simulink model "Verificacao_Controle_Pressao_2"  (R2018a)
settings: Solver=VariableStepAuto  StartTime=0.0  StopTime=60000  RelTol=1e-3
values from neighbouring files (symbols this model uses):
  alpha = Pacientes{i}('alpha')    [Analise_Exemplo.m]    (also in Analise_Geral_Robustez.m; Analise_Geral_Transitorio.m)
  Amplitude_perturbacao = 0    [Analise_Exemplo.m]    (also in Analise_Geral_Robustez.m = 25; Analise_Geral_Transitorio.m)
  ar = exp(-T/Constante_tempo_referencia)    [Analise_Exemplo.m]    (also in Analise_Geral_Robustez.m; Analise_Geral_Transitorio.m)
  ba_amplitude_seno = Pacientes{i}('ba_amplitude_seno')    [Analise_Exemplo.m]    (also in Analise_Geral_Robustez.m; Analise_Geral_Transitorio.m)
  ba_frequencia_seno = Pacientes{i}('ba_frequencia_seno')    [Analise_Exemplo.m]    (also in Analise_Geral_Robustez.m; Analise_Geral_Transitorio.m)
  ba_ganho_estocastico = Pacientes{i}('ba_ganho_estocastico')    [Analise_Exemplo.m]    (also in Analise_Geral_Robustez.m; Analise_Geral_Transitorio.m)
  ba_limiar_reflexo = Pacientes{i}('ba_limiar_reflexo')    [Analise_Exemplo.m]    (also in Analise_Geral_Robustez.m; Analise_Geral_Transitorio.m)
  ba_offset = Pacientes{i}('ba_offset')    [Analise_Exemplo.m]    (also in Analise_Geral_Robustez.m; Analise_Geral_Transitorio.m)
  comando_inicial = 0    [Analise_Exemplo.m]    (also in Analise_Geral_Robustez.m; Analise_Geral_Transitorio.m)
  d = 5    [Analise_Exemplo.m]    (also in Analise_Geral_Robustez.m; Analise_Geral_Transitorio.m)
  forgetting_factor = exp(-T/T_forgetting)    [Analise_Exemplo.m]    (also in Analise_Geral_Robustez.m; Analise_Geral_Transitorio.m)
  Instante_habilita_controlador = 30    [Analise_Exemplo.m]    (also in Analise_Geral_Robustez.m; Analise_Geral_Transitorio.m)
  Instante_habilita_perturbacao = 3*60*60    (= 10800)    [Analise_Exemplo.m]    (also in Analise_Geral_Robustez.m; Analise_Geral_Transitorio.m)
  K = Pacientes{i}('K')    [Analise_Exemplo.m]    (also in Analise_Geral_Robustez.m; Analise_Geral_Transitorio.m)
  P_inicial = [0.01 0 0; 0 0.001 0 ; 0 0 1]    [Analise_Exemplo.m]    (also in Analise_Geral_Robustez.m; Analise_Geral_Transitorio.m)
  saida_inicial_maxima = 0    [Analise_Exemplo.m]    (also in Analise_Geral_Robustez.m; Analise_Geral_Transitorio.m)
  semente_ruido = 2    [Analise_Exemplo.m]    (also in Analise_Geral_Robustez.m = j; Analise_Geral_Transitorio.m = j)
  setpoint_final = 116    [Analise_Exemplo.m]    (also in Analise_Geral_Robustez.m = 120; Analise_Geral_Transitorio.m)
  setpoint_inicial = 131    [Analise_Exemplo.m]    (also in Analise_Geral_Robustez.m = 150; Analise_Geral_Transitorio.m)
  T = 15    [Analise_Exemplo.m]    (also in Analise_Geral_Robustez.m; Analise_Geral_Transitorio.m)
  Tau = Pacientes{i}('Tau')    [Analise_Exemplo.m]    (also in Analise_Geral_Robustez.m; Analise_Geral_Transitorio.m)
  Tau_c = Pacientes{i}('Tau_c')    [Analise_Exemplo.m]    (also in Analise_Geral_Robustez.m; Analise_Geral_Transitorio.m)
  Tau_i = Pacientes{i}('Tau_i');5    [Analise_Exemplo.m]    (also in Analise_Geral_Robustez.m; Analise_Geral_Transitorio.m)
  Tempo_Segundo_Step = 30*60    (= 1800)    [Analise_Exemplo.m]    (also in Analise_Geral_Robustez.m; Analise_Geral_Transitorio.m)
  theta_inicial = [c0_inicial; c1_inicial; c2_inicial]    [Analise_Exemplo.m]    (also in Analise_Geral_Robustez.m; Analise_Geral_Transitorio.m)
libraries: simulink x1, powerlib_meascontrol x1
settings Model: Creator=gabri  LastModifiedBy=gabri

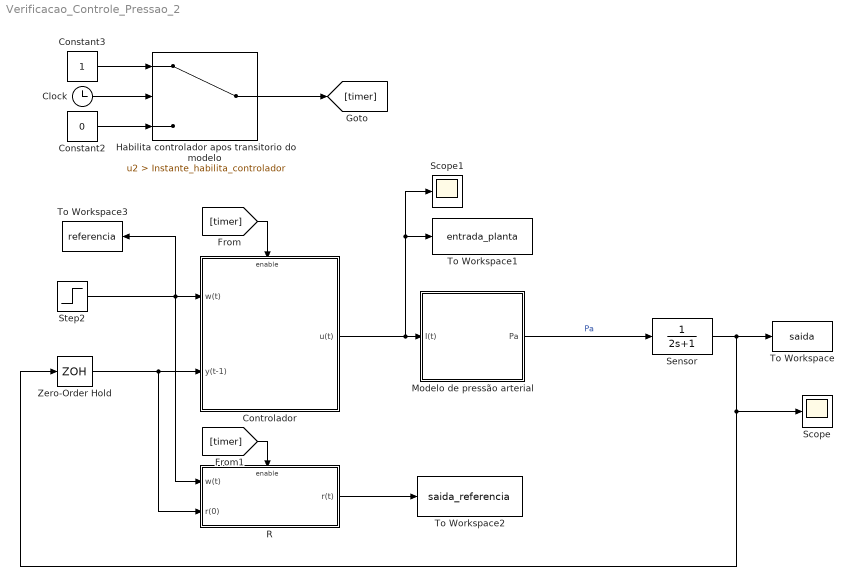
== system Verificacao_Controle_Pressao_2 ==
  Clock : Clock
  Constant2 : Constant  Value=0
  Constant3 : Constant
  "Controlador " : Subsystem
  Habilita controlador apos transitorio do modelo : Switch  Criteria=u2 > Threshold  Threshold=Instante_habilita_controlador  ZeroCross=off
  Modelo de pressão arterial : Subsystem
  R : Subsystem  TreatAsAtomicUnit=on
  Scope : Scope
  Scope1 : Scope
  Sensor : TransferFcn  Denominator=[2 1]
  Step2 : Step  Time=Instante_habilita_controlador+Tempo_Segundo_Step  Before=setpoint_inicial  After=setpoint_final  SampleTime=0
  To Workspace : ToWorkspace  VariableName=saida  SaveFormat=Timeseries  SampleTime=-1
  To Workspace1 : ToWorkspace  VariableName=entrada_planta  SaveFormat=Timeseries  SampleTime=-1
  To Workspace2 : ToWorkspace  VariableName=saida_referencia  SaveFormat=Timeseries  SampleTime=-1
  To Workspace3 : ToWorkspace  VariableName=referencia  SaveFormat=Timeseries  SampleTime=-1
  Zero-Order Hold : ZeroOrderHold  SampleTime=T
  wires:
  Constant2/1 -> Habilita controlador apos transitorio do modelo/3
  Habilita controlador apos transitorio do modelo/1 -> [timer]
  Clock/1 -> Habilita controlador apos transitorio do modelo/2
  Constant3/1 -> Habilita controlador apos transitorio do modelo/1
  Modelo de pressão arterial/1(Pa) -> Sensor/1  "Pa"
  [timer] -> "Controlador "/Enable
  R/1(r(t)) -> To Workspace2/1
  [timer] -> R/Enable
  Zero-Order Hold/1 -> R/2(r(0)), "Controlador "/2(y(t-1))
  "Controlador "/1(u(t)) -> Modelo de pressão arterial/1(I(t)), Scope1/1, To Workspace1/1
  Sensor/1 -> To Workspace/1, Scope/1, Zero-Order Hold/1
  Step2/1 -> R/1(w(t)), To Workspace3/1, "Controlador "/1(w(t))

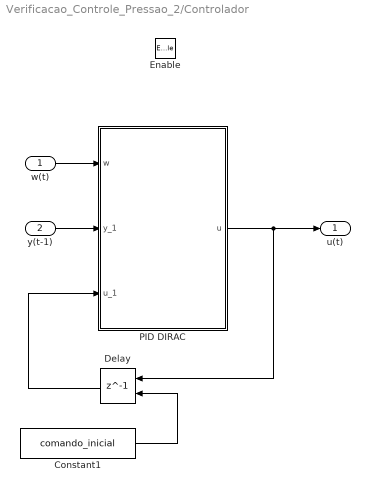
== system Verificacao_Controle_Pressao_2/Controlador  ==
  w(t) : Inport
  y(t-1) : Inport  Port=2
  Enable : EnablePort
  Constant1 : Constant  Value=comando_inicial
  Delay : Delay  DelayLength=1  InitialConditionSource=Input port  InitialCondition=0  SampleTime=T
      settings: InputPortMap=u0,p4
  PID DIRAC : Subsystem
  u(t) : Outport
  wires:
  w(t)/1 -> PID DIRAC/1("w ")
  Delay/1 -> PID DIRAC/3(u_1)
  y(t-1)/1 -> PID DIRAC/2(y_1)
  Constant1/1 -> Delay/2
  PID DIRAC/1(u) -> u(t)/1, Delay/1

== system Verificacao_Controle_Pressao_2/Modelo de pressão arterial ==
  I(t) : Inport
  Add : Sum
  Atividade de Background : Subsystem
  Resposta ao medicamento : Subsystem
  Pa : Outport
  wires:
  Resposta ao medicamento/1(Delta_Pd) -> Add/1
  I(t)/1 -> Resposta ao medicamento/1(I)
  Add/1 -> Pa/1, Atividade de Background/1(pa)  "Pa"
  Atividade de Background/1("Background Offset ") -> Add/2

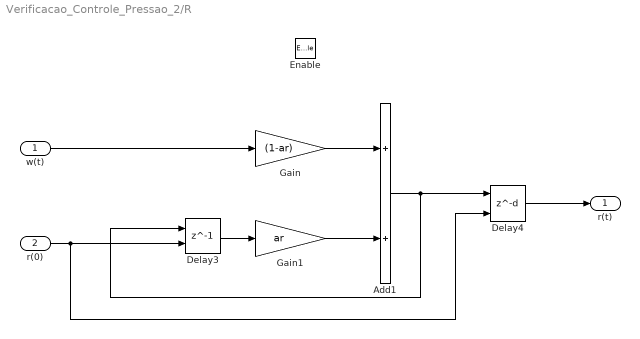
== system Verificacao_Controle_Pressao_2/R ==
  w(t) : Inport
  r(0) : Inport  Port=2
  Enable : EnablePort
  Add1 : Sum
  Delay3 : Delay  DelayLength=1  InitialConditionSource=Input port  InitialCondition=100  SampleTime=T
      settings: InputPortMap=u0,p4
  Delay4 : Delay  DelayLength=d  InitialConditionSource=Input port  InitialCondition=0  SampleTime=T
      settings: InputPortMap=u0,p4
  Gain : Gain  Gain=(1-ar)
  Gain1 : Gain  Gain=ar
  r(t) : Outport
  wires:
  Delay3/1 -> Gain1/1
  w(t)/1 -> Gain/1
  Gain1/1 -> Add1/2
  Gain/1 -> Add1/1
  r(0)/1 -> Delay4/2, Delay3/2
  Add1/1 -> Delay4/1, Delay3/1
  Delay4/1 -> r(t)/1

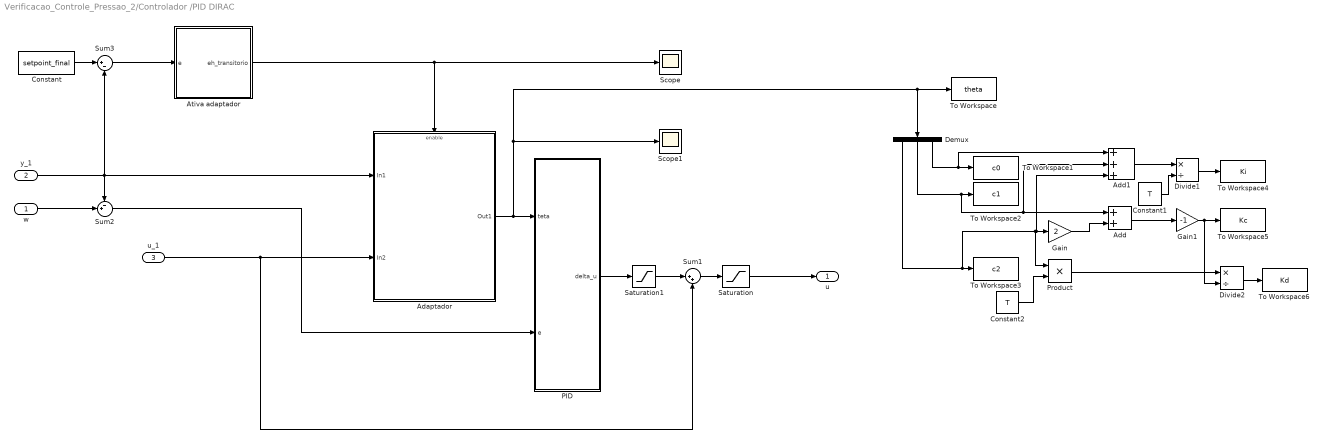
== system Verificacao_Controle_Pressao_2/Controlador /PID DIRAC ==
  "w " : Inport
  y_1 : Inport  Port=2
  u_1 : Inport  Port=3
  Adaptador : Subsystem
  Add : Sum
  Add1 : Sum  Inputs=+++
  Ativa adaptador : Subsystem
  Constant : Constant  Value=setpoint_final
  Constant1 : Constant  Value=T
  Constant2 : Constant  Value=T
  Demux : Demux  Outputs=3
  Divide1 : Product  Inputs=*/
  Divide2 : Product  Inputs=*/
  Gain : Gain  Gain=2
  Gain1 : Gain  Gain=-1
  PID : Subsystem
  Product : Product
  Saturation : Saturate  UpperLimit=180  LowerLimit=0
  Saturation1 : Saturate  UpperLimit=3  LowerLimit=-40
  Scope : Scope
  Scope1 : Scope
  Sum1 : Sum  Inputs=|++
  Sum2 : Sum  Inputs=-+|
  Sum3 : Sum  Inputs=|+-
  To Workspace : ToWorkspace  VariableName=theta  SaveFormat=Timeseries  SampleTime=-1
  To Workspace1 : ToWorkspace  VariableName=c0  SaveFormat=Timeseries  SampleTime=-1
  To Workspace2 : ToWorkspace  VariableName=c1  SaveFormat=Timeseries  SampleTime=-1
  To Workspace3 : ToWorkspace  VariableName=c2  SaveFormat=Timeseries  SampleTime=-1
  To Workspace4 : ToWorkspace  VariableName=Ki  SaveFormat=Timeseries  SampleTime=-1
  To Workspace5 : ToWorkspace  VariableName=Kc  SaveFormat=Timeseries  SampleTime=-1
  To Workspace6 : ToWorkspace  VariableName=Kd  SaveFormat=Timeseries  SampleTime=-1
  u : Outport
  wires:
  PID/1(delta_u) -> Saturation1/1
  Sum1/1 -> Saturation/1
  Saturation1/1 -> Sum1/1
  Saturation/1 -> u/1
  Sum2/1 -> PID/2(e)
  "w "/1 -> Sum2/2
  u_1/1 -> Sum1/2, Adaptador/2(In2)
  Constant/1 -> Sum3/1
  y_1/1 -> Adaptador/1(In1), Sum3/2, Sum2/1
  Ativa adaptador/1(eh_transitorio) -> Adaptador/Enable, Scope/1
  Sum3/1 -> Ativa adaptador/1(e)
  Demux/3 -> Add1/1, To Workspace1/1
  Demux/1 -> Product/1, Add1/3, Gain/1, To Workspace3/1
  Demux/2 -> Add1/2, Add/1, To Workspace2/1
  Adaptador/1(Out1) -> Scope1/1, To Workspace/1, Demux/1, PID/1(teta)
  Gain/1 -> Add/2
  Add/1 -> Gain1/1
  Add1/1 -> Divide1/1
  Constant1/1 -> Divide1/2
  Constant2/1 -> Product/2
  Product/1 -> Divide2/1
  Divide1/1 -> To Workspace4/1
  Gain1/1 -> Divide2/2, To Workspace5/1
  Divide2/1 -> To Workspace6/1

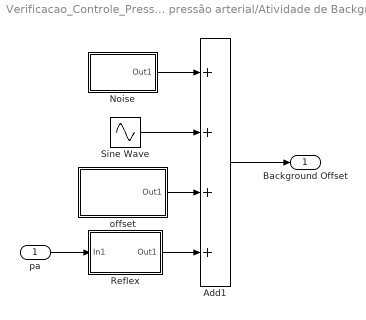
== system Verificacao_Controle_Pressao_2/Modelo de pressão arterial/Atividade de Background ==
  pa : Inport
  Add1 : Sum  Inputs=++++
  "Noise " : Subsystem
  Reflex : Subsystem
  Sine Wave : Sin  Amplitude=ba_amplitude_seno  Frequency=ba_frequencia_seno  SampleTime=0
  offset : Subsystem
  "Background Offset " : Outport
  wires:
  Reflex/1(Out1) -> Add1/4
  Add1/1 -> "Background Offset "/1
  "Noise "/1(Out1) -> Add1/1
  Sine Wave/1 -> Add1/2
  pa/1 -> Reflex/1(In1)
  offset/1(Out1) -> Add1/3

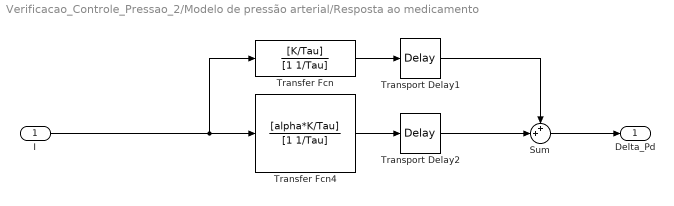
== system Verificacao_Controle_Pressao_2/Modelo de pressão arterial/Resposta ao medicamento ==
  I : Inport
  Sum : Sum  Inputs=++|
  Transfer Fcn : TransferFcn  Numerator=[K/Tau]  Denominator=[1 1/Tau]
  Transfer Fcn4 : TransferFcn  Numerator=[alpha*K/Tau]  Denominator=[1 1/Tau]
  Transport Delay1 : TransportDelay  DelayTime=Tau_i
  Transport Delay2 : TransportDelay  DelayTime=Tau_i+Tau_c
  Delta_Pd : Outport
  wires:
  Transport Delay1/1 -> Sum/1
  I/1 -> Transfer Fcn/1, Transfer Fcn4/1
  Transfer Fcn/1 -> Transport Delay1/1
  Transfer Fcn4/1 -> Transport Delay2/1
  Transport Delay2/1 -> Sum/2
  Sum/1 -> Delta_Pd/1

== system Verificacao_Controle_Pressao_2/Controlador /PID DIRAC/Adaptador ==
  In1 : Inport
  In2 : Inport  Port=2
  Enable : EnablePort
  Estimador2 : Subsystem
  Interface do Estimador : Subsystem
  Out1 : Outport
  wires:
  In1/1 -> Interface do Estimador/1("yf(t) ")
  Estimador2/1(theta) -> Out1/1
  Interface do Estimador/1("psi ") -> Estimador2/1(psi)
  Interface do Estimador/2(phi) -> Estimador2/2(phi)
  In2/1 -> Interface do Estimador/2(uf(t))

== system Verificacao_Controle_Pressao_2/Controlador /PID DIRAC/Ativa adaptador ==
  e : Inport
  Constant1 : Constant  Value=0
  Constant3 : Constant
  Is accomodated after rising : Subsystem
  Switch1 : Switch  Threshold=1
  eh_transitorio : Outport
  wires:
  Switch1/1 -> eh_transitorio/1
  e/1 -> Is accomodated after rising/1(In1)
  Is accomodated after rising/1(Out1) -> Switch1/2
  Constant3/1 -> Switch1/3
  Constant1/1 -> Switch1/1

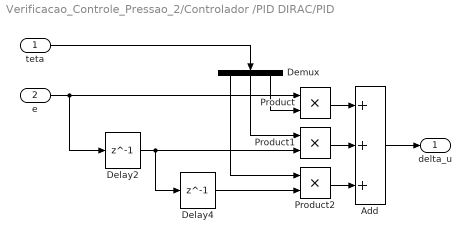
== system Verificacao_Controle_Pressao_2/Controlador /PID DIRAC/PID ==
  teta : Inport
  e : Inport  Port=2
  Add : Sum  Inputs=+++
  Delay2 : Delay  DelayLength=1  InitialCondition=0  SampleTime=T
  Delay4 : Delay  DelayLength=1  InitialCondition=0  SampleTime=T
  Demux : Demux  Outputs=3
  Product : Product
  Product1 : Product
  Product2 : Product
  delta_u : Outport
  wires:
  teta/1 -> Demux/1
  Delay2/1 -> Product1/2, Delay4/1
  Delay4/1 -> Product2/2
  Add/1 -> delta_u/1
  Demux/3 -> Product/2
  Demux/2 -> Product1/1
  Demux/1 -> Product2/1
  Product/1 -> Add/1
  Product1/1 -> Add/2
  Product2/1 -> Add/3
  e/1 -> Delay2/1, Product/1

== system Verificacao_Controle_Pressao_2/Modelo de pressão arterial/Atividade de Background/Noise  ==
  Random Number : RandomNumber  Seed=semente_ruido  SampleTime=T
  Saturation : Saturate  UpperLimit=ba_ganho_estocastico  LowerLimit=-ba_ganho_estocastico
  Transfer Fcn : TransferFcn  Numerator=[ba_ganho_estocastico]  Denominator=[30^2 2*30 1]
  Out1 : Outport
  wires:
  Transfer Fcn/1 -> Saturation/1
  Random Number/1 -> Transfer Fcn/1
  Saturation/1 -> Out1/1

== system Verificacao_Controle_Pressao_2/Modelo de pressão arterial/Atividade de Background/Reflex ==
  In1 : Inport
  Add2 : Sum  Inputs=-+
  Constant2 : Constant  Value=ba_limiar_reflexo
  Saturation : Saturate  UpperLimit=0  LowerLimit=-35
  Transfer Fcn2 : TransferFcn  Denominator=[240 1]
  Transport Delay : TransportDelay  DelayTime=40
  Out1 : Outport
  wires:
  Saturation/1 -> Transport Delay/1
  In1/1 -> Add2/2
  Transport Delay/1 -> Transfer Fcn2/1
  Constant2/1 -> Add2/1
  Add2/1 -> Saturation/1
  Transfer Fcn2/1 -> Out1/1

== system Verificacao_Controle_Pressao_2/Modelo de pressão arterial/Atividade de Background/offset ==
  Constant2 : Constant  Value=ba_offset
  Step : Step  Time=Instante_habilita_perturbacao  After=Amplitude_perturbacao  SampleTime=0
  Sum1 : Sum  Inputs=++|
  To Workspace : ToWorkspace  VariableName=atividade_background  SaveFormat=Timeseries  SampleTime=-1
  Out1 : Outport
  wires:
  Constant2/1 -> Sum1/1
  Step/1 -> Sum1/2
  Sum1/1 -> To Workspace/1, Out1/1

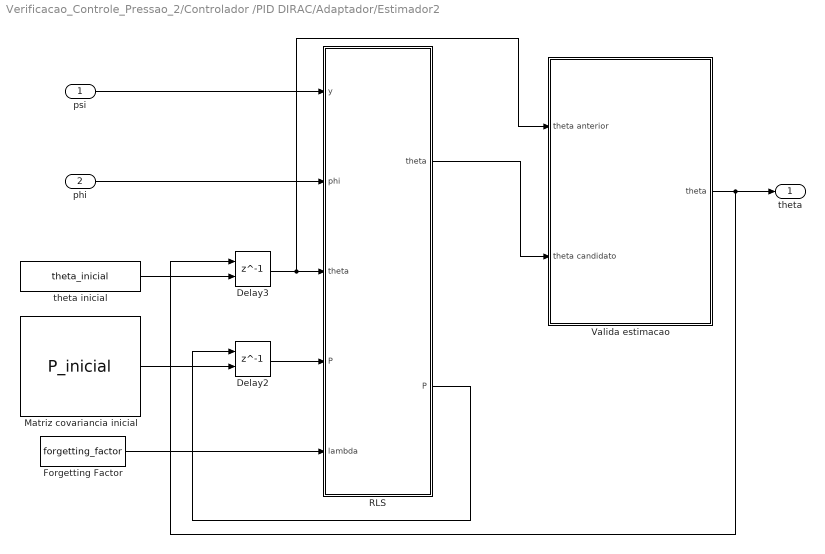
== system Verificacao_Controle_Pressao_2/Controlador /PID DIRAC/Adaptador/Estimador2 ==
  psi : Inport
  phi : Inport  Port=2
  Delay2 : Delay  DelayLength=1  InitialConditionSource=Input port  InitialCondition=0  SampleTime=T
      settings: InputPortMap=u0,p4
  Delay3 : Delay  DelayLength=1  InitialConditionSource=Input port  InitialCondition=0  SampleTime=T
      settings: InputPortMap=u0,p4
  Forgetting Factor : Constant  Value=forgetting_factor
  Matriz covariancia inicial : Constant  Value=P_inicial
  RLS : MATLAB Function  TreatAsAtomicUnit=on
  Valida estimacao : Subsystem
  theta inicial : Constant  Value=theta_inicial
  theta : Outport
  wires:
  Delay3/1 -> Valida estimacao/1(theta anterior), RLS/3("theta ")
  RLS/1(theta) -> Valida estimacao/2(theta candidato)
  Valida estimacao/1(theta) -> Delay3/1, theta/1
  Forgetting Factor/1 -> RLS/5(lambda)
  psi/1 -> RLS/1(y)
  RLS/2(P) -> Delay2/1
  theta inicial/1 -> Delay3/2
  phi/1 -> RLS/2(phi)
  Delay2/1 -> RLS/4("P ")
  Matriz covariancia inicial/1 -> Delay2/2

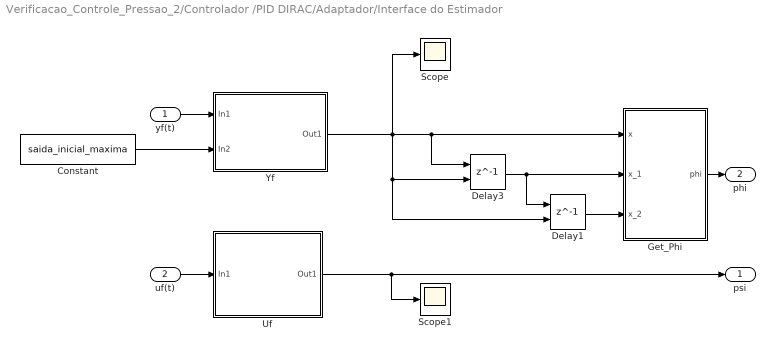
== system Verificacao_Controle_Pressao_2/Controlador /PID DIRAC/Adaptador/Interface do Estimador ==
  "yf(t) " : Inport
  uf(t) : Inport  Port=2
  Constant : Constant  Value=saida_inicial_maxima
  Delay1 : Delay  DelayLength=1  InitialConditionSource=Input port  InitialCondition=0  SampleTime=T
      settings: InputPortMap=u0,p4
  Delay3 : Delay  DelayLength=1  InitialConditionSource=Input port  InitialCondition=0  SampleTime=T
      settings: InputPortMap=u0,p4
  "Get_Phi " : MATLAB Function  TreatAsAtomicUnit=on
  Scope : Scope
  Scope1 : Scope
  Uf : Subsystem
  Yf : Subsystem
  "psi " : Outport
  phi : Outport  Port=2
  wires:
  Delay1/1 -> "Get_Phi "/3(x_2)
  Delay3/1 -> "Get_Phi "/2(x_1), Delay1/1
  "Get_Phi "/1(phi) -> phi/1
  Yf/1(Out1) -> Delay1/2, Delay3/2, Scope/1, Delay3/1, "Get_Phi "/1(x)
  Uf/1(Out1) -> Scope1/1, "psi "/1
  Constant/1 -> Yf/2(In2)
  "yf(t) "/1 -> Yf/1(In1)
  uf(t)/1 -> Uf/1(In1)

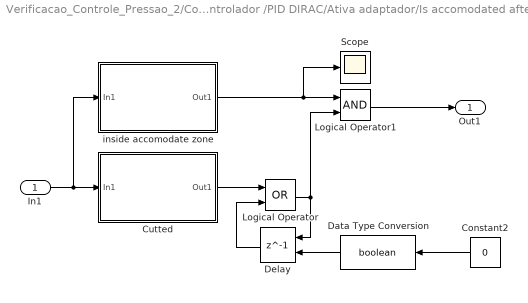
== system Verificacao_Controle_Pressao_2/Controlador /PID DIRAC/Ativa adaptador/Is accomodated after rising ==
  In1 : Inport
  Constant2 : Constant  Value=0
  Cutted : Subsystem
  Data Type Conversion : DataTypeConversion  OutDataTypeStr=boolean
  Delay : Delay  DelayLength=1  InitialConditionSource=Input port  InitialCondition=0
      settings: InputPortMap=u0,p4
  Logical Operator : Logic  Operator=OR  AllPortsSameDT=off  OutDataTypeStr=boolean
  Logical Operator1 : Logic  AllPortsSameDT=off  OutDataTypeStr=boolean
  Scope : Scope
  inside accomodate zone : Subsystem
  Out1 : Outport
  wires:
  inside accomodate zone/1(Out1) -> Scope/1, Logical Operator1/1
  Logical Operator/1 -> Logical Operator1/2, Delay/1
  Constant2/1 -> Data Type Conversion/1
  Logical Operator1/1 -> Out1/1
  In1/1 -> inside accomodate zone/1(In1), Cutted/1(In1)
  Cutted/1(Out1) -> Logical Operator/1
  Delay/1 -> Logical Operator/2
  Data Type Conversion/1 -> Delay/2

== system Verificacao_Controle_Pressao_2/Controlador /PID DIRAC/Adaptador/Estimador2/Valida estimacao ==
  theta anterior : Inport
  theta candidato : Inport  Port=2
  Compare To Zero : simulink/Logic and Bit Operations/Compare To Zero  relop=<=  OutDataTypeStr=boolean
  Switch2 : Switch  Criteria=u2 > Threshold
  Valida Estimacao : MATLAB Function  TreatAsAtomicUnit=on
  theta : Outport
  wires:
  Switch2/1 -> theta/1
  Compare To Zero/1 -> Switch2/2
  theta anterior/1 -> Switch2/3
  Valida Estimacao/1(eh_invalido) -> Compare To Zero/1
  theta candidato/1 -> Switch2/1, Valida Estimacao/1(theta_candidato)

== system Verificacao_Controle_Pressao_2/Controlador /PID DIRAC/Adaptador/Interface do Estimador/Uf ==
  In1 : Inport
  Delay2 : Delay  DelayLength=1
  R : Subsystem  TreatAsAtomicUnit=on
  Sum3 : Sum  Inputs=|+-
  Out1 : Outport
  wires:
  R/1(r(t)) -> Sum3/1, Delay2/1
  Delay2/1 -> Sum3/2
  Sum3/1 -> Out1/1
  In1/1 -> R/2(r(0)), R/1(w(t))

== system Verificacao_Controle_Pressao_2/Controlador /PID DIRAC/Adaptador/Interface do Estimador/Yf ==
  In1 : Inport
  In2 : Inport  Port=2
  R : Subsystem  TreatAsAtomicUnit=on
  Sum2 : Sum  Inputs=|+-
  Sum4 : Sum  Inputs=|-+
  Out1 : Outport
  wires:
  Sum4/1 -> Out1/1
  In2/1 -> Sum2/2
  R/1(r(t)) -> Sum4/1
  In1/1 -> Sum2/1
  Sum2/1 -> R/1(w(t)), R/2(r(0)), Sum4/2

== system Verificacao_Controle_Pressao_2/Controlador /PID DIRAC/Ativa adaptador/Is accomodated after rising/Cutted ==
  In1 : Inport
  Constant2 : Constant  Value=0
  Edge Detector : powerlib_meascontrol/Logic/Edge Detector  model=Rising  ic=0  Ts=0
      settings: SourceProductName=Simscape Power Systems  SourceProductBaseCode=PS
  Relational Operator : RelationalOperator  Operator=>  OutDataTypeStr=boolean  RndMeth=Simplest
  Out1 : Outport
  wires:
  Constant2/1 -> Relational Operator/2
  Relational Operator/1 -> Edge Detector/1
  In1/1 -> Relational Operator/1
  Edge Detector/1 -> Out1/1

== system Verificacao_Controle_Pressao_2/Controlador /PID DIRAC/Ativa adaptador/Is accomodated after rising/inside accomodate zone ==
  In1 : Inport
  Abs1 : Abs
  Constant3 : Constant  Value=10
  Relational Operator1 : RelationalOperator  Operator=<  OutDataTypeStr=boolean  RndMeth=Simplest
  Out1 : Outport
  wires:
  Constant3/1 -> Relational Operator1/2
  Relational Operator1/1 -> Out1/1
  In1/1 -> Abs1/1
  Abs1/1 -> Relational Operator1/1

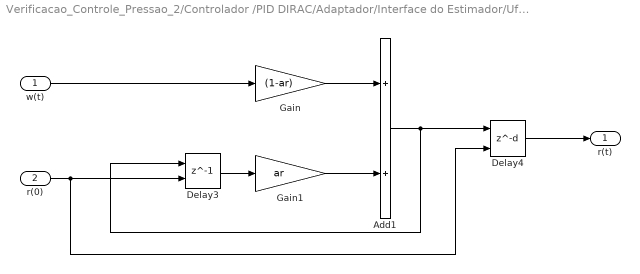
== system Verificacao_Controle_Pressao_2/Controlador /PID DIRAC/Adaptador/Interface do Estimador/Uf/R ==
  w(t) : Inport
  r(0) : Inport  Port=2
  Add1 : Sum
  Delay3 : Delay  DelayLength=1  InitialConditionSource=Input port  InitialCondition=100  SampleTime=T
      settings: InputPortMap=u0,p4
  Delay4 : Delay  DelayLength=d  InitialConditionSource=Input port  InitialCondition=0  SampleTime=T
      settings: InputPortMap=u0,p4
  Gain : Gain  Gain=(1-ar)
  Gain1 : Gain  Gain=ar
  r(t) : Outport
  wires:
  Delay3/1 -> Gain1/1
  w(t)/1 -> Gain/1
  Gain1/1 -> Add1/2
  Gain/1 -> Add1/1
  r(0)/1 -> Delay4/2, Delay3/2
  Add1/1 -> Delay4/1, Delay3/1
  Delay4/1 -> r(t)/1

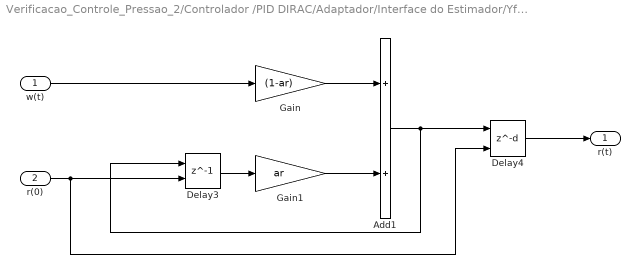
== system Verificacao_Controle_Pressao_2/Controlador /PID DIRAC/Adaptador/Interface do Estimador/Yf/R ==
  w(t) : Inport
  r(0) : Inport  Port=2
  Add1 : Sum
  Delay3 : Delay  DelayLength=1  InitialConditionSource=Input port  InitialCondition=100  SampleTime=T
      settings: InputPortMap=u0,p4
  Delay4 : Delay  DelayLength=d  InitialConditionSource=Input port  InitialCondition=0  SampleTime=T
      settings: InputPortMap=u0,p4
  Gain : Gain  Gain=(1-ar)
  Gain1 : Gain  Gain=ar
  r(t) : Outport
  wires:
  Delay3/1 -> Gain1/1
  w(t)/1 -> Gain/1
  Gain1/1 -> Add1/2
  Gain/1 -> Add1/1
  r(0)/1 -> Delay4/2, Delay3/2
  Add1/1 -> Delay4/1, Delay3/1
  Delay4/1 -> r(t)/1

== matlab function Verificacao_Controle_Pressao_2/Controlador /PID DIRAC/Adaptador/Estimador2/Valida estimacao/Valida Estimacao ==
  data: theta_candidato input; eh_invalido output
function eh_invalido  = fcn(theta_candidato)
    c0 = theta_candidato(1);
    c1 = theta_candidato(2);
    c2 = theta_candidato(3);

    eh_invalido = 1;
    %if(c0<0 && c1>0 && c2<0)
    %    eh_invalido = 0;
    %end
    T = 15;
    Kc = -(c1+2*c2);
    Ti = -T*(c1+2*c2)/(c0+c1+c2);
    Td = -T*c2/(c1+2*c2);
    
    if(Kc<0 && Ti>0 && Td>0)
        eh_invalido = 0;
    end
    
end

== matlab function Verificacao_Controle_Pressao_2/Controlador /PID DIRAC/Adaptador/Estimador2/RLS ==
  data: theta output; y input; phi input; theta input; P input; P output; lambda input
function [theta, P] = fcn(y, phi, theta, P, lambda)
    E = y - theta.'*phi;
    P = (P - (P*(phi*phi.')*P)/(lambda+phi.'*P*phi))/lambda;
    theta = theta + P*phi*E;
end

== matlab function Verificacao_Controle_Pressao_2/Controlador /PID DIRAC/Adaptador/Interface do Estimador/Get_Phi  ==
  data: x input; x_1 input; phi output; x_2 input
function phi = fcn(x, x_1, x_2)
    phi = [x; x_1; x_2];
end
